simulink model "RuntimeDAC1"  (R2017b)
settings: Solver=FixedStepDiscrete  StartTime=0.0  StopTime=10.0  FixedStep=1e-4  RelTol=1e-3
libraries: mbed_lib x5, simulink x1
settings Model: Creator=oh  LastModifiedBy=oh
settings DataIOCC: LimitDataPoints=on  SaveFormat=Array  ReturnWorkspaceOutputs=on  LoggingToFile=on
settings OptimizationCC: DefaultParameterBehavior=Inlined
settings DebuggingCC: ParameterTunabilityLossMsg=error  SFUnexpectedBacktrackingDiag=warning  SFNoUnconditionalDefaultTransitionDiag=warning  SFExecutionAtInitializationDiag=none
settings HardwareCC: ProdBitPerPointer=32  ProdBitPerSizeT=32  ProdBitPerPtrDiffT=32  ProdLargestAtomicInteger=Long  ProdLargestAtomicFloat=Double  ProdWordSize=32  ProdHWDeviceType=ARM Compatible->ARM Cortex
settings ModelReferenceCC: PropagateSignalLabelsOutOfModel=off
settings SFSimCC: MATLABDynamicMemAlloc=off
settings RTWCC: SystemTargetFile=mbed.tlc  TemplateMakefile=mbed.tmf  Description=MbedTarget (Embedded Target for Embedded Coder)  IncludeHyperlinkInReport=on  TargetLang=C++
settings CodeAppCC: ForceParamTrailComments=on  IgnoreCustomStorageClasses=off  OperatorAnnotations=on  SimulinkDataObjDesc=on  SFDataObjDesc=on  MATLABFcnDesc=on  InsertBlockDesc=on  StateflowObjectComments=on  MATLABSourceComments=on
settings STFCustomTargetCC: TargetLibSuffix=.a  GenerateSampleERTMain=on  CombineOutputUpdateFcns=on  ERTCustomFileBanners=on  SupportNonInlinedSFcns=off  RemoveResetFunc=on  MATLABClassNameForMDSCustomization=Simulink.SoftwareTarget.ERTCustomization  ModelStepFunctionPrototypeControlCompliant=on  GRTInterface=off  SystemTargetFile=mbed.tlc
settings ERTTargetCC: MultiwordLength=2048  GenerateSampleERTMain=on  ParMdlRefBuildCompliant=off  CompOptLevelCompliant=off  ConcurrentExecutionCompliant=off  SupportContinuousTime=on  CPPClassGenCompliant=off  UseToolchainInfoCompliant=off  InlinedParameterPlacement=NonHierarchical  ERTCustomFileTemplate=mbed_file_process.tlc
settings ConfigComp: CovMetricSettings=dw  CovHtmlReporting=on  CovSaveCumulativeToWorkspaceVar=on  CovSaveSingleToWorkspaceVar=on  CovExternalEMLEnable=off

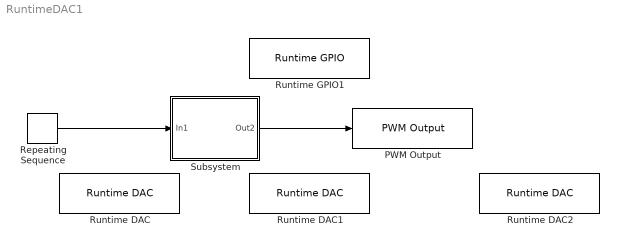
== system RuntimeDAC1 ==
  PWM Output : mbed_lib/GPIO/PWM Output  Priority=4  PortName=B  PinNumber=11  Period=1000  SampleTime=-1
      settings: SourceProductName=Mbed Target
  Repeating Sequence : simulink/Sources/Repeating Sequence  Priority=0  rep_seq_t=[0 2]  rep_seq_y=[0 2*pi]
  Runtime DAC : mbed_lib/GPIO/Runtime DAC  PortName=A  PinNumber=4  Mode=Set Value  DacValue=0.1  SampleTime=-1
      settings: SourceProductName=Mbed Target
  Runtime DAC1 : mbed_lib/GPIO/Runtime DAC  PortName=A  PinNumber=4  Mode=Set Value  DacValue=0.5  SampleTime=-1
      settings: SourceProductName=Mbed Target
  Runtime DAC2 : mbed_lib/GPIO/Runtime DAC  PortName=A  PinNumber=4  Mode=Set Value  DacValue=0  SampleTime=-1
      settings: SourceProductName=Mbed Target
  Runtime GPIO1 : mbed_lib/GPIO/Runtime GPIO  PortName=A  PinNumber=0  SampleTime=-1
      settings: SourceProductName=Mbed Target
  Subsystem : Subsystem  Priority=2  TreatAsAtomicUnit=on
  wires:
  Repeating Sequence/1 -> Subsystem/1(In1)
  Subsystem/1(Out2) -> PWM Output/1

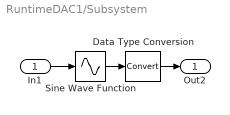
== system RuntimeDAC1/Subsystem ==
  In1 : Inport
  Data Type Conversion : DataTypeConversion
  Sine Wave Function : Sin  TimeSource=Use external signal  SampleTime=0
  Out2 : Outport
  wires:
  In1/1 -> Sine Wave Function/1
  Sine Wave Function/1 -> Data Type Conversion/1
  Data Type Conversion/1 -> Out2/1
